simulink model "call_stats_bolck1"  (R2018a)
settings: Solver=VariableStepAuto  StartTime=0.0  StopTime=10.0  RelTol=1e-3
settings Model: Creator=jdrjk  LastModifiedBy=jdrjk

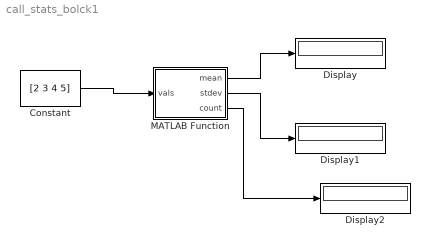
== system call_stats_bolck1 ==
  Constant : Constant  Value=[2 3 4 5]
  Display : Display
  Display1 : Display
  Display2 : Display
  MATLAB Function : MATLAB Function  TreatAsAtomicUnit=on  SystemSampleTime=0.1
  wires:
  Constant/1 -> MATLAB Function/1(vals)
  MATLAB Function/1(mean) -> Display/1
  MATLAB Function/2(stdev) -> Display1/1
  MATLAB Function/3(count) -> Display2/1

== matlab function call_stats_bolck1/MATLAB Function ==
  data: vals input; mean output; stdev output; count output
function [mean,stdev,count] = stats(vals)

persistent count1;
if(isempty(count1))
    count1 = 0;
end

count1 = count1 + 1;
count = count1;
len = length(vals);
mean = avg(vals,len);
stdev = sqrt(sum(((vals-avg(vals,len)).^2))/len);
plot(vals,'-+');

function mean = avg(array,size)
mean = sum(array)/size;
